simulink model "wave_superposition"  (R2021b)
settings: Solver=VariableStepAuto  StartTime=0.0  StopTime=10.0  RelTol=1e-3
settings Model: Creator=admin  LastModifiedBy=admin

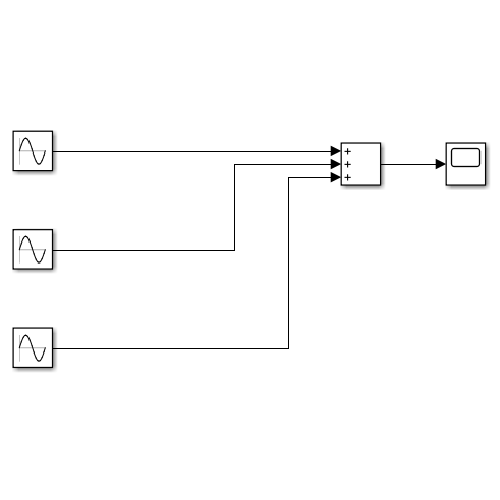
[thumbnail: Simulink's stored preview of the top-level diagram]
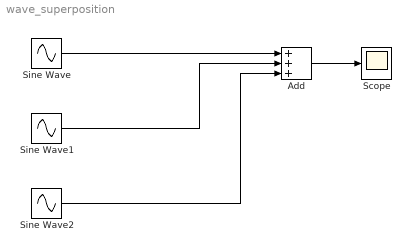
== system wave_superposition ==
  Add : Sum  Inputs=+++
  Scope : Scope
  Sine Wave : Sin  SampleTime=0
  Sine Wave1 : Sin  Amplitude=0.5  Frequency=3  SampleTime=0
  Sine Wave2 : Sin  Amplitude=0.3  Frequency=5  SampleTime=0
  wires:
  Sine Wave/1 -> Add/1
  Sine Wave1/1 -> Add/2
  Add/1 -> Scope/1
  Sine Wave2/1 -> Add/3
